simulink model "laterl_model_esp"  (R2020a)
settings: Solver=ode45  StartTime=0.0  StopTime=Tfinal  RelTol=1e-3  EnableMultiTasking=on
undefined symbols (not defined in the file): Calpha, Cf, Cr, Izz, K, Ke, l, lf, lr, m, mu, SteerAngle, Tc, Vx_const, Vy0, X0, Y0, Yaw0, yaw_rate0
settings Model: Creator=user  LastModifiedBy=USER
settings SolverCC: ZeroCrossAlgorithm=Non-adaptive
settings DataIOCC: LimitDataPoints=on  SaveFormat=Array  SignalLoggingSaveFormat=ModelDataLogs  ReturnWorkspaceOutputs=off
settings OptimizationCC: ExpressionDepthLimit=2147483647  InitFltsAndDblsToZero=on  LifeSpan=inf
settings DebuggingCC: UnderspecifiedInitializationDetection=Classic  MergeDetectMultiDrivingBlocksExec=none  SolverPrmCheckMsg=warning  FcnCallInpInsideContextMsg=warning  StateNameClashWarn=warning  SFUnexpectedBacktrackingDiag=warning  SFNoUnconditionalDefaultTransitionDiag=warning  SFExecutionAtInitializationDiag=none  ArithmeticOperatorsInVariantConditions=warning
settings HardwareCC: ProdBitPerPointer=32  ProdBitPerSizeT=32  ProdBitPerPtrDiffT=32  ProdLargestAtomicFloat=None  ProdIntDivRoundTo=Undefined  ProdEndianess=Unspecified  ProdWordSize=32  ProdHWDeviceType=32-bit Generic
settings ModelReferenceCC: PropagateSignalLabelsOutOfModel=off
settings CodeAppCC: StateflowObjectComments=on
settings GRTTargetCC: TargetLangStandard=C89/C90 (ANSI)  CombineOutputUpdateFcns=off  GRTInterface=on
settings ConfigComp: CovMetricSettings=dw  CovHtmlReporting=on  CovSaveCumulativeToWorkspaceVar=on  CovSaveSingleToWorkspaceVar=on

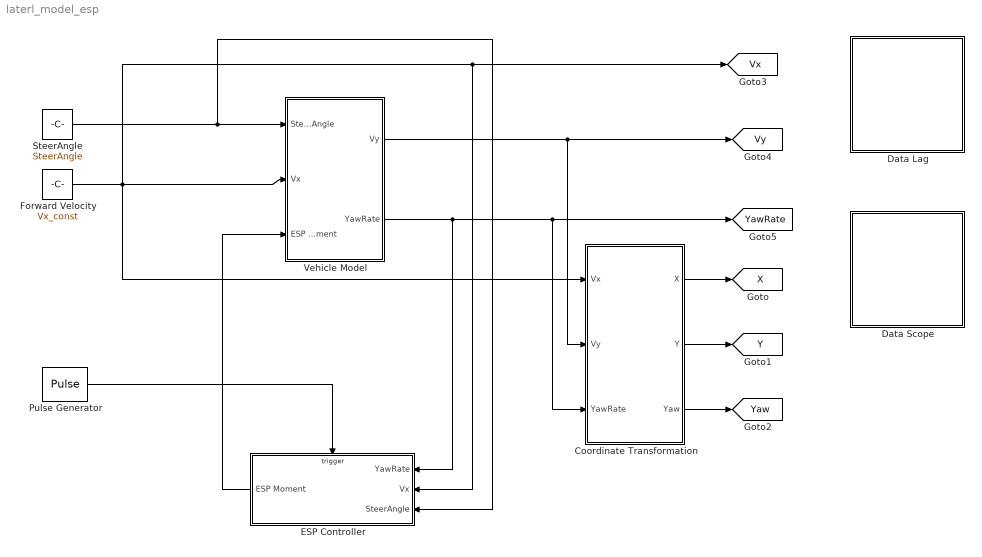
== system laterl_model_esp ==
  Coordinate Transformation : Subsystem
  Data Lag : Subsystem
  Data Scope : Subsystem
  ESP Controller : Subsystem
  Forward Velocity : Constant  Value=Vx_const
  Pulse Generator : DiscretePulseGenerator  PulseType=Time based  Period=Tc  PulseWidth=50
  SteerAngle : Constant  Value=SteerAngle
  Vehicle Model : Subsystem
  tag scope: Vx=global, Vy=global, X=global, Y=global, Yaw=global, YawRate=global
  wires:
  SteerAngle/1 -> Vehicle Model/1(Steering_Angle), ESP Controller/3(SteerAngle)
  Forward Velocity/1 -> Vehicle Model/2(Vx), Coordinate Transformation/1(Vx), [Vx], ESP Controller/2(Vx)
  Vehicle Model/1(Vy) -> Coordinate Transformation/2(Vy), [Vy]
  Vehicle Model/2(YawRate) -> Coordinate Transformation/3(YawRate), [YawRate], ESP Controller/1(YawRate)
  Coordinate Transformation/1(X) -> [X]
  Coordinate Transformation/2(Y) -> [Y]
  Coordinate Transformation/3(Yaw) -> [Yaw]
  ESP Controller/1(ESP Moment) -> Vehicle Model/3(ESP Moment)
  Pulse Generator/1 -> ESP Controller/Trigger

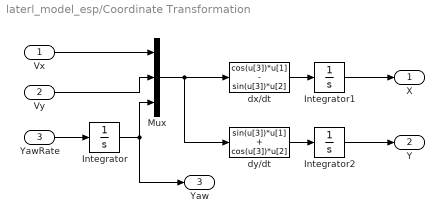
== system laterl_model_esp/Coordinate Transformation ==
  Vx : Inport
  Vy : Inport  Port=2
  YawRate : Inport  Port=3
  Integrator : Integrator  InitialCondition=Yaw0
  Integrator1 : Integrator  InitialCondition=X0
  Integrator2 : Integrator  InitialCondition=Y0
  Mux : Mux  Inputs=3
  dx/dt : Fcn  Expr=cos(u[3])*u[1] - sin(u[3])*u[2]
  dy/dt : Fcn  Expr=sin(u[3])*u[1] + cos(u[3])*u[2]
  X : Outport
  Y : Outport  Port=2
  Yaw : Outport  Port=3
  wires:
  YawRate/1 -> Integrator/1
  Vx/1 -> Mux/1
  Vy/1 -> Mux/2
  Integrator/1 -> Mux/3, Yaw/1
  Mux/1 -> dx/dt/1, dy/dt/1
  dx/dt/1 -> Integrator1/1
  Integrator1/1 -> X/1
  dy/dt/1 -> Integrator2/1
  Integrator2/1 -> Y/1

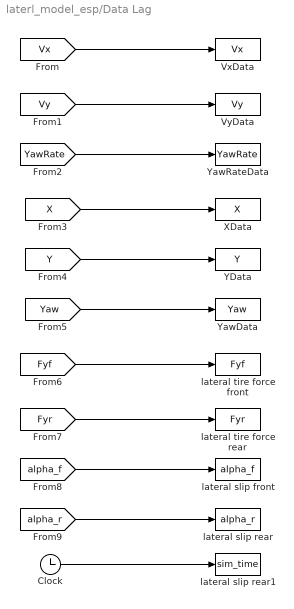
== system laterl_model_esp/Data Lag ==
  Clock : Clock
  VxData : ToWorkspace  VariableName=Vx  SampleTime=-1
  VyData : ToWorkspace  VariableName=Vy  SampleTime=-1
  XData : ToWorkspace  VariableName=X  SampleTime=-1
  YData : ToWorkspace  VariableName=Y  SampleTime=-1
  YawData : ToWorkspace  VariableName=Yaw  SampleTime=-1
  YawRateData : ToWorkspace  VariableName=YawRate  SampleTime=-1
  lateral slip front : ToWorkspace  VariableName=alpha_f  SampleTime=-1
  lateral slip rear : ToWorkspace  VariableName=alpha_r  SampleTime=-1
  lateral slip rear1 : ToWorkspace  VariableName=sim_time  SampleTime=-1
  lateral tire force front : ToWorkspace  VariableName=Fyf  SampleTime=-1
  lateral tire force rear : ToWorkspace  VariableName=Fyr  SampleTime=-1
  wires:
  [Vx] -> VxData/1
  [Vy] -> VyData/1
  [YawRate] -> YawRateData/1
  [X] -> XData/1
  [Y] -> YData/1
  [Yaw] -> YawData/1
  [Fyf] -> lateral tire force front/1
  [Fyr] -> lateral tire force rear/1
  [alpha_f] -> lateral slip front/1
  [alpha_r] -> lateral slip rear/1
  Clock/1 -> lateral slip rear1/1

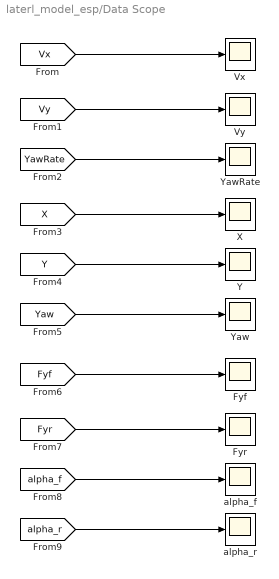
== system laterl_model_esp/Data Scope ==
  Fyf : Scope
  Fyr : Scope
  Vx : Scope
  Vy : Scope
  X : Scope
  Y : Scope
  Yaw : Scope
  YawRate : Scope
  alpha_f : Scope
  alpha_r : Scope
  wires:
  [Vx] -> Vx/1
  [Vy] -> Vy/1
  [YawRate] -> YawRate/1
  [X] -> X/1
  [Y] -> Y/1
  [Yaw] -> Yaw/1
  [Fyf] -> Fyf/1
  [Fyr] -> Fyr/1
  [alpha_f] -> alpha_f/1
  [alpha_r] -> alpha_r/1

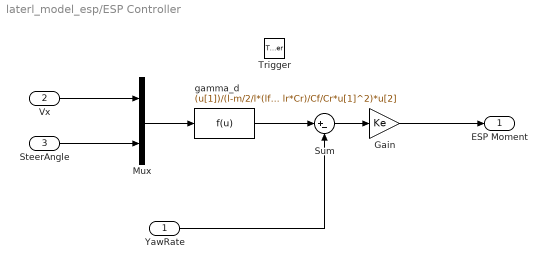
== system laterl_model_esp/ESP Controller ==
  YawRate : Inport
  Vx : Inport  Port=2
  SteerAngle : Inport  Port=3
  Trigger : TriggerPort  VariantControl=(inherit)
  Gain : Gain  Gain=Ke
  Mux : Mux  Inputs=2
  Sum : Sum  Inputs=|+-
  gamma_d : Fcn  Expr=(u[1])/(l-m/2/l*(lf*Cf - lr*Cr)/Cf/Cr*u[1]^2)*u[2]
  ESP Moment : Outport
  wires:
  Vx/1 -> Mux/1
  SteerAngle/1 -> Mux/2
  Mux/1 -> gamma_d/1
  gamma_d/1 -> Sum/1
  YawRate/1 -> Sum/2
  Sum/1 -> Gain/1
  Gain/1 -> ESP Moment/1

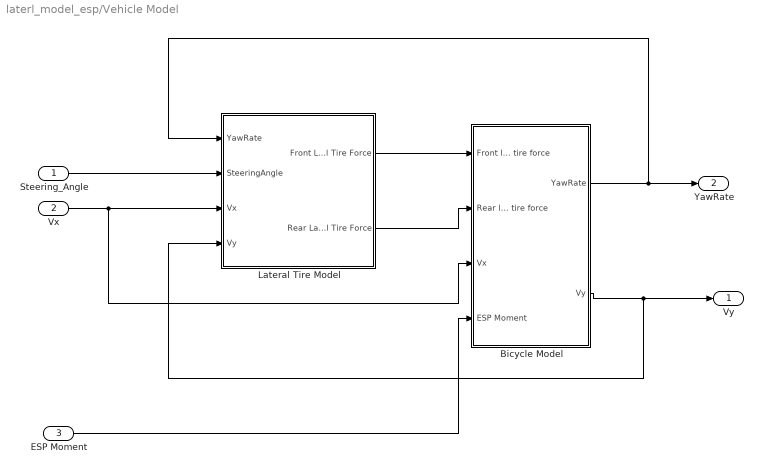
== system laterl_model_esp/Vehicle Model ==
  Steering_Angle : Inport
  Vx : Inport  Port=2
  ESP Moment : Inport  Port=3
  Bicycle Model : Subsystem
  Lateral Tire Model : Subsystem
  Vy : Outport
  YawRate : Outport  Port=2
  wires:
  Steering_Angle/1 -> Lateral Tire Model/2(SteeringAngle)
  Lateral Tire Model/1(Front Lateral Tire Force) -> Bicycle Model/1(Front lateral tire force)
  Lateral Tire Model/2(Rear Lateral Tire Force) -> Bicycle Model/2(Rear lateral tire force)
  Bicycle Model/1(YawRate) -> Lateral Tire Model/1(YawRate), YawRate/1
  Bicycle Model/2(Vy) -> Vy/1, Lateral Tire Model/4(Vy)
  Vx/1 -> Lateral Tire Model/3(Vx), Bicycle Model/3(Vx)
  ESP Moment/1 -> Bicycle Model/4(ESP Moment)

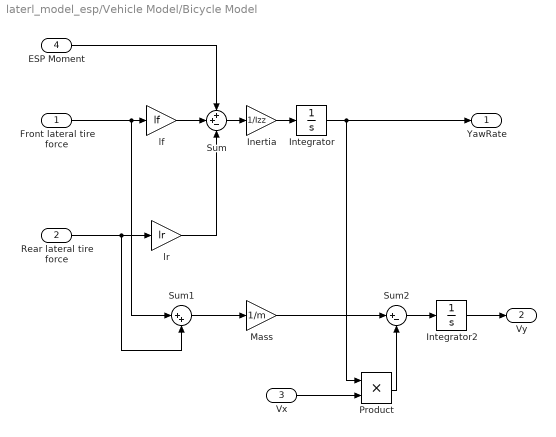
== system laterl_model_esp/Vehicle Model/Bicycle Model ==
  Front lateral tire force : Inport
  Rear lateral tire force : Inport  Port=2
  Vx : Inport  Port=3
  ESP Moment : Inport  Port=4
  Inertia : Gain  Gain=1/Izz
  Integrator : Integrator  InitialCondition=yaw_rate0
  Integrator2 : Integrator  InitialCondition=Vy0
  Mass : Gain  Gain=1/m
  Product : Product  RndMeth=Zero
  Sum : Sum  Inputs=++-
  Sum1 : Sum  Inputs=|++
  Sum2 : Sum  Inputs=|+-
  lf : Gain  Gain=lf
  lr : Gain  Gain=lr
  YawRate : Outport
  Vy : Outport  Port=2
  wires:
  Front lateral tire force/1 -> lf/1, Sum1/1
  Rear lateral tire force/1 -> lr/1, Sum1/2
  Sum/1 -> Inertia/1
  Inertia/1 -> Integrator/1
  Integrator/1 -> YawRate/1, Product/1
  Sum1/1 -> Mass/1
  Mass/1 -> Sum2/1
  Vx/1 -> Product/2
  Product/1 -> Sum2/2
  Sum2/1 -> Integrator2/1
  Integrator2/1 -> Vy/1
  ESP Moment/1 -> Sum/1
  lf/1 -> Sum/2
  lr/1 -> Sum/3

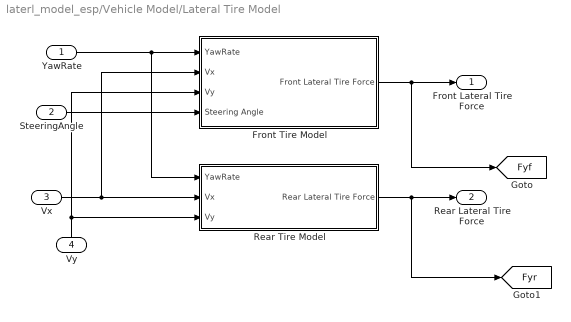
== system laterl_model_esp/Vehicle Model/Lateral Tire Model ==
  YawRate : Inport
  SteeringAngle : Inport  Port=2
  Vx : Inport  Port=3
  Vy : Inport  Port=4
  Front Tire Model : Subsystem
  Rear Tire Model : Subsystem
  Front Lateral Tire Force : Outport
  Rear Lateral Tire Force : Outport  Port=2
  tag scope: Fyf=global, Fyr=global
  wires:
  Vx/1 -> Rear Tire Model/2(Vx), Front Tire Model/2(Vx)
  Vy/1 -> Rear Tire Model/3(Vy), Front Tire Model/3(Vy)
  YawRate/1 -> Front Tire Model/1(YawRate), Rear Tire Model/1(YawRate)
  Front Tire Model/1(Front Lateral Tire Force) -> Front Lateral Tire Force/1, [Fyf]
  SteeringAngle/1 -> Front Tire Model/4(Steering Angle)
  Rear Tire Model/1(Rear Lateral Tire Force) -> Rear Lateral Tire Force/1, [Fyr]

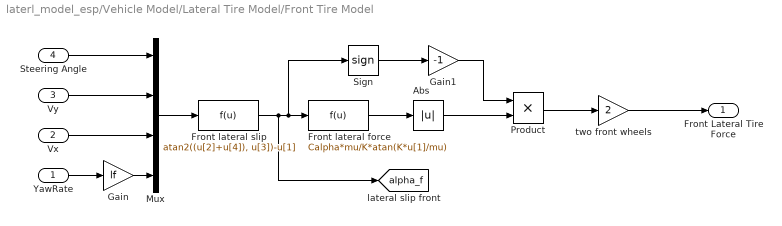
== system laterl_model_esp/Vehicle Model/Lateral Tire Model/Front Tire Model ==
  YawRate : Inport
  Vx : Inport  Port=2
  Vy : Inport  Port=3
  Steering Angle : Inport  Port=4
  Abs : Abs
  Front lateral force : Fcn  Expr=Calpha*mu/K*atan(K*u[1]/mu)
  Front lateral slip : Fcn  Expr=atan2((u[2]+u[4]), u[3])-u[1]
  Gain : Gain  Gain=lf
  Gain1 : Gain  Gain=-1
  Mux : Mux
  Product : Product  RndMeth=Zero
  Sign : Signum
  two front wheels : Gain  Gain=2
  Front Lateral Tire Force : Outport
  tag scope: alpha_f=global
  wires:
  Steering Angle/1 -> Mux/1
  Vy/1 -> Mux/2
  Vx/1 -> Mux/3
  YawRate/1 -> Gain/1
  Mux/1 -> Front lateral slip/1
  Gain/1 -> Mux/4
  Front lateral slip/1 -> [alpha_f], Front lateral force/1, Sign/1
  Front lateral force/1 -> Abs/1
  Sign/1 -> Gain1/1
  Gain1/1 -> Product/1
  Abs/1 -> Product/2
  Product/1 -> two front wheels/1
  two front wheels/1 -> Front Lateral Tire Force/1

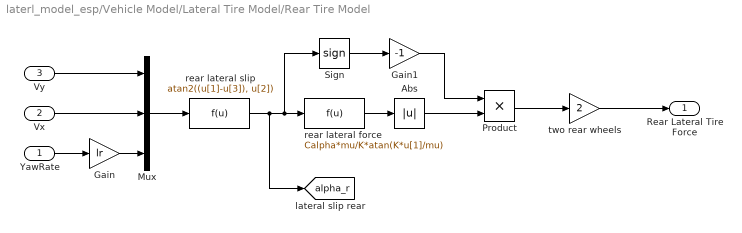
== system laterl_model_esp/Vehicle Model/Lateral Tire Model/Rear Tire Model ==
  YawRate : Inport
  Vx : Inport  Port=2
  Vy : Inport  Port=3
  Abs : Abs
  Gain : Gain  Gain=lr
  Gain1 : Gain  Gain=-1
  Mux : Mux  Inputs=3
  Product : Product  RndMeth=Zero
  Sign : Signum
  rear lateral force : Fcn  Expr=Calpha*mu/K*atan(K*u[1]/mu)
  rear lateral slip : Fcn  Expr=atan2((u[1]-u[3]), u[2])
  two rear wheels : Gain  Gain=2
  Rear Lateral Tire Force : Outport
  tag scope: alpha_r=global
  wires:
  rear lateral slip/1 -> [alpha_r], rear lateral force/1, Sign/1
  Gain/1 -> Mux/3
  Mux/1 -> rear lateral slip/1
  YawRate/1 -> Gain/1
  Vy/1 -> Mux/1
  Vx/1 -> Mux/2
  Sign/1 -> Gain1/1
  rear lateral force/1 -> Abs/1
  Gain1/1 -> Product/1
  Abs/1 -> Product/2
  Product/1 -> two rear wheels/1
  two rear wheels/1 -> Rear Lateral Tire Force/1
